simulink model "Agent_ZP_Mananger"  (R2018a)
settings: Solver=FixedStepAuto  StartTime=0.0  StopTime=Inf  FixedStep=0.0000001  RelTol=1e-3
(part 1 of 2)
settings Model: Creator=lenovo  LastModifiedBy=lenovo

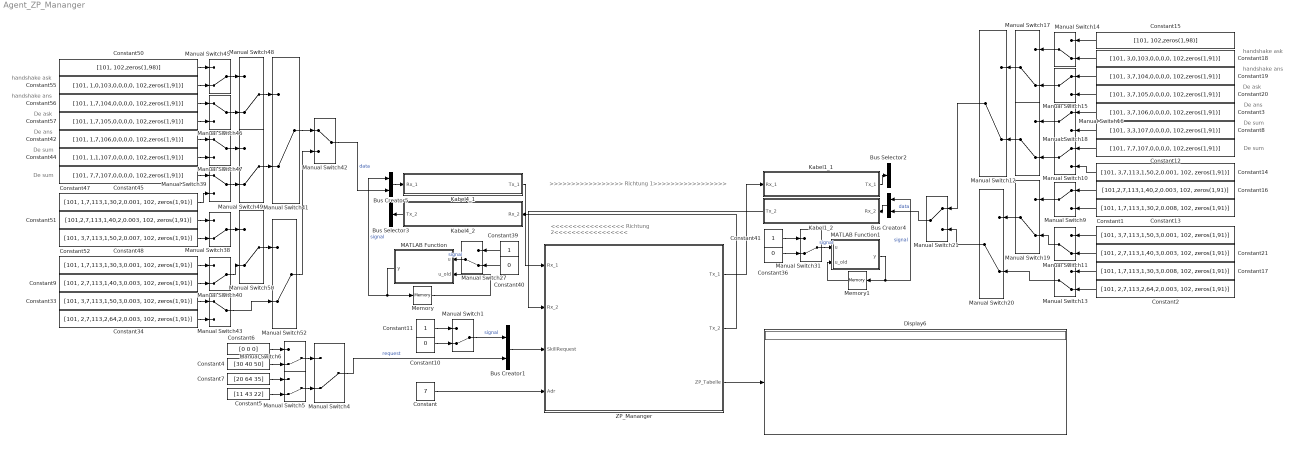
== system Agent_ZP_Mananger ==
  note: >>>>>>>>>>>>>>>>> Richtung 1>>>>>>>>>>>>>>>>>
  note: handshake ask
  note: De sum
  note: handshake ans
  note: De ask
  note: De ans
  note: De sum
  note: De ask
  note: De sum
  note: De ans
  note: handshake ans
  note: De sum
  note: handshake ask
  note: <<<<<<<<<<<<<<<<< Richtung 2<<<<<<<<<<<<<<<<<
  Bus Creator1 : BusCreator  Inputs=2
  Bus Creator4 : BusCreator  Inputs=2
  Bus Creator5 : BusCreator  Inputs=2
  Bus Selector2 : BusSelector  OutputSignals=signal,data
  Bus Selector3 : BusSelector  OutputSignals=signal,data
  Constant : Constant  Value=7  OutDataTypeStr=double
  Constant1 : Constant  Value=[101, 3,7,113,1,50,3,0.001, 102, zeros(1,91)]  OutDataTypeStr=double
  Constant10 : Constant  Value=0  OutDataTypeStr=boolean
  Constant11 : Constant  OutDataTypeStr=boolean
  Constant12 : Constant  Value=[101, 7,7,107,0,0,0,0, 102,zeros(1,91)]  OutDataTypeStr=double
  Constant13 : Constant  Value=[101, 1,7,113,1,30,2,0.008, 102, zeros(1,91)]  OutDataTypeStr=double
  Constant14 : Constant  Value=[101, 3,7,113,1,50,2,0.001, 102, zeros(1,91)]  OutDataTypeStr=double
  Constant15 : Constant  Value=[101, 102,zeros(1,98)]  OutDataTypeStr=double
  Constant16 : Constant  Value=[101,2,7,113,1,40,2,0.003, 102, zeros(1,91)]  OutDataTypeStr=double
  Constant17 : Constant  Value=[101, 1,7,113,1,30,3,0.008, 102, zeros(1,91)]  OutDataTypeStr=double
  Constant18 : Constant  Value=[101, 3,0,103,0,0,0,0, 102,zeros(1,91)]  OutDataTypeStr=double
  Constant19 : Constant  Value=[101, 3,7,104,0,0,0,0, 102,zeros(1,91)]  OutDataTypeStr=double
  Constant2 : Constant  Value=[101, 2,7,113,2,64,2,0.003, 102, zeros(1,91)]  OutDataTypeStr=double
  Constant20 : Constant  Value=[101, 3,7,105,0,0,0,0, 102,zeros(1,91)]  OutDataTypeStr=double
  Constant21 : Constant  Value=[101, 2,7,113,1,40,3,0.003, 102, zeros(1,91)]  OutDataTypeStr=double
  Constant3 : Constant  Value=[101, 3,7,106,0,0,0,0, 102,zeros(1,91)]  OutDataTypeStr=double
  Constant33 : Constant  Value=[101, 3,7,113,1,50,3,0.003, 102, zeros(1,91)]  OutDataTypeStr=double
  Constant34 : Constant  Value=[101, 2,7,113,2,64,2,0.003, 102, zeros(1,91)]  OutDataTypeStr=double
  Constant36 : Constant  Value=0  OutDataTypeStr=boolean
  Constant39 : Constant  OutDataTypeStr=boolean
  Constant4 : Constant  Value=[30 40 50]
  Constant40 : Constant  Value=0  OutDataTypeStr=boolean
  Constant41 : Constant  OutDataTypeStr=boolean
  Constant42 : Constant  Value=[101, 1,7,106,0,0,0,0, 102,zeros(1,91)]  OutDataTypeStr=double
  Constant44 : Constant  Value=[101, 1,1,107,0,0,0,0, 102,zeros(1,91)]  OutDataTypeStr=double
  Constant45 : Constant  Value=[101, 7,7,107,0,0,0,0, 102,zeros(1,91)]  OutDataTypeStr=double
  Constant47 : Constant  Value=[101, 1,7,113,1,30,2,0.001, 102, zeros(1,91)]  OutDataTypeStr=double
  Constant48 : Constant  Value=[101, 3,7,113,1,50,2,0.007, 102, zeros(1,91)]  OutDataTypeStr=double
  Constant5 : Constant  Value=[11 43 22]
  Constant50 : Constant  Value=[101, 102,zeros(1,98)]  OutDataTypeStr=double
  Constant51 : Constant  Value=[101,2,7,113,1,40,2,0.003, 102, zeros(1,91)]  OutDataTypeStr=double
  Constant52 : Constant  Value=[101, 1,7,113,1,30,3,0.001, 102, zeros(1,91)]  OutDataTypeStr=double
  Constant55 : Constant  Value=[101, 1,0,103,0,0,0,0, 102,zeros(1,91)]  OutDataTypeStr=double
  Constant56 : Constant  Value=[101, 1,7,104,0,0,0,0, 102,zeros(1,91)]  OutDataTypeStr=double
  Constant57 : Constant  Value=[101, 1,7,105,0,0,0,0, 102,zeros(1,91)]  OutDataTypeStr=double
  Constant6 : Constant  Value=[0 0 0]
  Constant7 : Constant  Value=[20 64 35]
  Constant8 : Constant  Value=[101, 3,3,107,0,0,0,0, 102,zeros(1,91)]  OutDataTypeStr=double
  Constant9 : Constant  Value=[101, 2,7,113,1,40,3,0.003, 102, zeros(1,91)]  OutDataTypeStr=double
  Display6 : Display
  Kabel1_1 : Subsystem  TreatAsAtomicUnit=on
  Kabel1_2 : Subsystem  TreatAsAtomicUnit=on
  Kabel4_1 : Subsystem  TreatAsAtomicUnit=on
  Kabel4_2 : Subsystem  TreatAsAtomicUnit=on
  MATLAB Function : MATLAB Function  TreatAsAtomicUnit=on  SystemSampleTime=0.00001
  MATLAB Function1 : MATLAB Function  TreatAsAtomicUnit=on  SystemSampleTime=0.00001
  Manual Switch{1,4..6,11..14,17..20,27,31,38,40..41,45,48..50,52} (22 alike) : ManualSwitch  CurrentSetting=0
  Manual Switch{9..10,15..16,21,39,42..43,46..47} (10 alike) : ManualSwitch
  Memory : Memory  InitialCondition=false
  Memory1 : Memory  InitialCondition=false
  ZP_Mananger : Subsystem
  wires:
  Constant4/1 -> Manual Switch6/2
  Constant7/1 -> Manual Switch5/1
  Constant6/1 -> Manual Switch6/1
  Constant5/1 -> Manual Switch5/2
  Manual Switch5/1 -> Manual Switch4/2
  Manual Switch6/1 -> Manual Switch4/1
  Constant40/1 -> Manual Switch27/2
  Kabel1_1/1(Tx_1) -> Bus Selector2/1
  MATLAB Function/1(y) -> Memory/1, Bus Creator5/1  "signal"
  Bus Creator5/1 -> Kabel4_1/1(Rx_1)
  Bus Creator4/1 -> Kabel1_2/1(Rx_2)
  Constant36/1 -> Manual Switch31/2
  Constant41/1 -> Manual Switch31/1
  Memory1/1 -> MATLAB Function1/2(u_old)
  Manual Switch31/1 -> MATLAB Function1/1(u)  "signal"
  Memory/1 -> MATLAB Function/2(u_old)
  Manual Switch27/1 -> MATLAB Function/1(u)  "signal"
  MATLAB Function1/1(y) -> Bus Creator4/1, Memory1/1  "signal"
  Constant39/1 -> Manual Switch27/1
  Kabel4_2/1(Tx_2) -> Bus Selector3/1
  Constant44/1 -> Manual Switch47/2
  Constant57/1 -> Manual Switch46/2
  Constant56/1 -> Manual Switch46/1
  Constant55/1 -> Manual Switch45/2
  Constant50/1 -> Manual Switch45/1
  Manual Switch52/1 -> Manual Switch42/2
  Manual Switch50/1 -> Manual Switch52/1
  Manual Switch47/1 -> Manual Switch49/1
  Manual Switch38/1 -> Manual Switch50/1
  Manual Switch43/1 -> Manual Switch52/2
  Manual Switch48/1 -> Manual Switch41/1
  Constant42/1 -> Manual Switch47/1
  Manual Switch39/1 -> Manual Switch49/2
  Manual Switch46/1 -> Manual Switch48/2
  Manual Switch49/1 -> Manual Switch41/2
  Manual Switch45/1 -> Manual Switch48/1
  Manual Switch41/1 -> Manual Switch42/1
  Constant45/1 -> Manual Switch39/1
  Manual Switch40/1 -> Manual Switch50/2
  Manual Switch42/1 -> Bus Creator5/2  "data"
  Manual Switch21/1 -> Bus Creator4/2  "data"
  Constant47/1 -> Manual Switch39/2
  Constant51/1 -> Manual Switch38/1
  Constant48/1 -> Manual Switch38/2
  Constant52/1 -> Manual Switch40/1
  Constant9/1 -> Manual Switch40/2
  Constant33/1 -> Manual Switch43/1
  Constant34/1 -> Manual Switch43/2
  Constant20/1 -> Manual Switch15/2
  Manual Switch10/1 -> Manual Switch18/2
  Constant3/1 -> Manual Switch16/1
  Constant1/1 -> Manual Switch11/1
  Manual Switch17/1 -> Manual Switch12/1
  Manual Switch16/1 -> Manual Switch18/1
  Manual Switch19/1 -> Manual Switch20/1
  Constant15/1 -> Manual Switch14/1
  Constant18/1 -> Manual Switch14/2
  Manual Switch15/1 -> Manual Switch17/2
  Manual Switch18/1 -> Manual Switch12/2
  Manual Switch14/1 -> Manual Switch17/1
  Manual Switch11/1 -> Manual Switch19/2
  Constant8/1 -> Manual Switch16/2
  Constant12/1 -> Manual Switch10/1
  Constant21/1 -> Manual Switch11/2
  Manual Switch9/1 -> Manual Switch19/1
  Constant2/1 -> Manual Switch13/2
  Constant19/1 -> Manual Switch15/1
  Manual Switch13/1 -> Manual Switch20/2
  Constant16/1 -> Manual Switch9/1
  Manual Switch12/1 -> Manual Switch21/1
  Manual Switch20/1 -> Manual Switch21/2
  Constant13/1 -> Manual Switch9/2
  Constant14/1 -> Manual Switch10/2
  Constant17/1 -> Manual Switch13/1
  Kabel4_1/1(Tx_1) -> ZP_Mananger/1(Rx_1)
  Kabel1_2/1(Tx_2) -> ZP_Mananger/2(Rx_2)
  Constant/1 -> ZP_Mananger/4(Adr)
  ZP_Mananger/1(Tx_1) -> Kabel1_1/1(Rx_1)
  ZP_Mananger/2(Tx_2) -> Kabel4_2/1(Rx_2)
  Manual Switch1/1 -> Bus Creator1/1  "signal"
  Manual Switch4/1 -> Bus Creator1/2  "request"
  Bus Creator1/1 -> ZP_Mananger/3(SkillRequest)
  Constant10/1 -> Manual Switch1/2
  Constant11/1 -> Manual Switch1/1
  ZP_Mananger/3(ZP_Tabelle) -> Display6/1

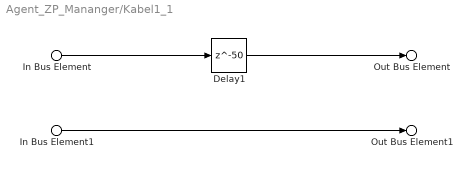
== system Agent_ZP_Mananger/Kabel1_1 ==
  In Bus Element : Inport  PortName=Rx_1  Element=signal
  In Bus Element1 : Inport  PortName=Rx_1  Element=data
  Delay1 : Delay  DelayLength=50
  Out Bus Element : Outport  PortName=Tx_1  Element=signal
  Out Bus Element1 : Outport  PortName=Tx_1  Element=data
  wires:
  In Bus Element/1 -> Delay1/1
  Delay1/1 -> Out Bus Element/1
  In Bus Element1/1 -> Out Bus Element1/1

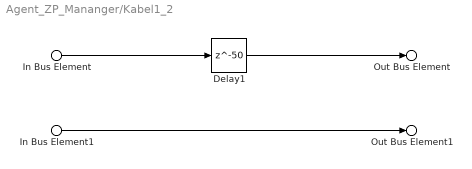
== system Agent_ZP_Mananger/Kabel1_2 ==
  In Bus Element : Inport  PortName=Rx_2  Element=signal
  In Bus Element1 : Inport  PortName=Rx_2  Element=data
  Delay1 : Delay  DelayLength=50
  Out Bus Element : Outport  PortName=Tx_2  Element=signal
  Out Bus Element1 : Outport  PortName=Tx_2  Element=data
  wires:
  In Bus Element/1 -> Delay1/1
  Delay1/1 -> Out Bus Element/1
  In Bus Element1/1 -> Out Bus Element1/1

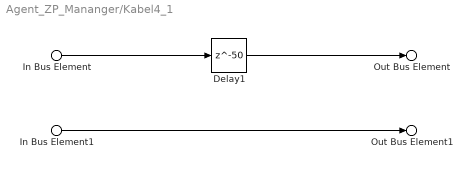
== system Agent_ZP_Mananger/Kabel4_1 ==
  In Bus Element : Inport  PortName=Rx_1  Element=signal
  In Bus Element1 : Inport  PortName=Rx_1  Element=data
  Delay1 : Delay  DelayLength=50
  Out Bus Element : Outport  PortName=Tx_1  Element=signal
  Out Bus Element1 : Outport  PortName=Tx_1  Element=data
  wires:
  In Bus Element/1 -> Delay1/1
  Delay1/1 -> Out Bus Element/1
  In Bus Element1/1 -> Out Bus Element1/1

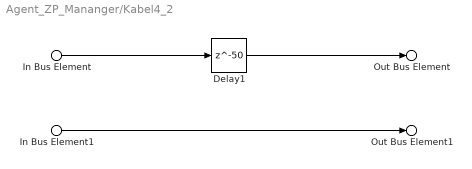
== system Agent_ZP_Mananger/Kabel4_2 ==
  In Bus Element : Inport  PortName=Rx_2  Element=signal
  In Bus Element1 : Inport  PortName=Rx_2  Element=data
  Delay1 : Delay  DelayLength=50
  Out Bus Element : Outport  PortName=Tx_2  Element=signal
  Out Bus Element1 : Outport  PortName=Tx_2  Element=data
  wires:
  In Bus Element/1 -> Delay1/1
  Delay1/1 -> Out Bus Element/1
  In Bus Element1/1 -> Out Bus Element1/1

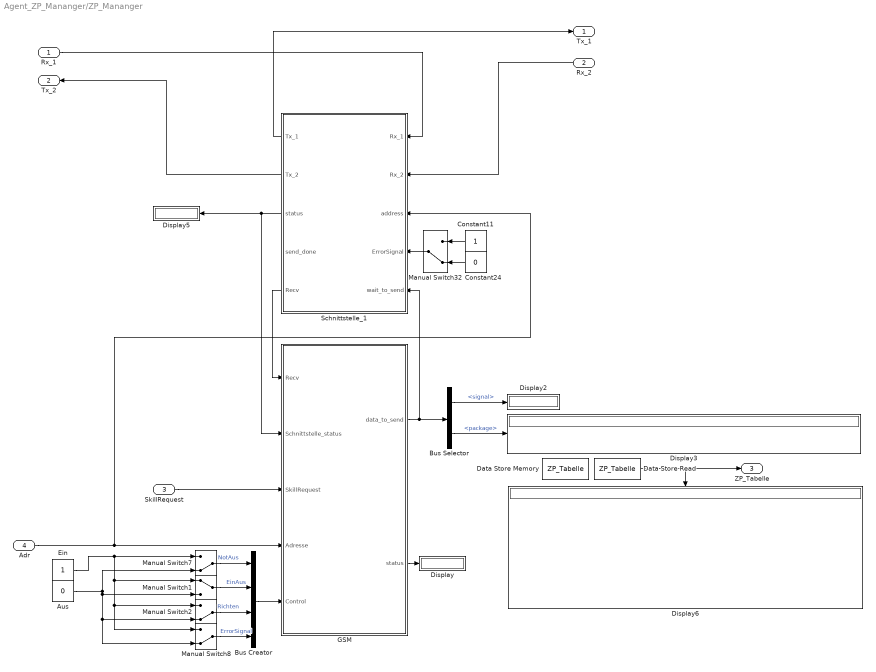
== system Agent_ZP_Mananger/ZP_Mananger ==
  Rx_1 : Inport
  Rx_2 : Inport  Port=2
  SkillRequest : Inport  Port=3
  Adr : Inport  Port=4
  Aus : Constant  Value=0  OutDataTypeStr=boolean
  Bus Creator : BusCreator  Inputs=4
  Bus Selector : BusSelector  OutputSignals=signal,package
  Constant11 : Constant  OutDataTypeStr=boolean
  Constant24 : Constant  Value=0  OutDataTypeStr=boolean
  Data Store Memory : DataStoreMemory  DataStoreName=ZP_Tabelle  ReadBeforeWriteMsg=warning  WriteAfterWriteMsg=warning  WriteAfterReadMsg=warning  InitialValue=zeros(10,7)  ShowAdditionalParam=off  OutDataTypeStr=double  Dimensions=[10 7]
  Data Store Read : DataStoreRead  DataStoreName=ZP_Tabelle
  Display{,2..3,5..6} (5 alike) : Display
  Ein : Constant  OutDataTypeStr=boolean
  "GSM " : Subsystem
  Manual Switch1 : ManualSwitch
  Manual Switch{2,7..8,32} (4 alike) : ManualSwitch  CurrentSetting=0
  Schnittstelle_1 : Subsystem
  Tx_1 : Outport
  Tx_2 : Outport  Port=2
  ZP_Tabelle : Outport  Port=3
  wires:
  Bus Selector/1 -> Display2/1  "<signal>"
  Ein/1 -> Manual Switch7/1, Manual Switch1/1, Manual Switch2/1, Manual Switch8/1
  Data Store Read/1 -> ZP_Tabelle/1, Display6/1
  Schnittstelle_1/5(Recv) -> "GSM "/1(Recv)
  Aus/1 -> Manual Switch7/2, Manual Switch1/2, Manual Switch2/2, Manual Switch8/2
  Manual Switch32/1 -> Schnittstelle_1/4(ErrorSignal)
  Manual Switch1/1 -> Bus Creator/2  "EinAus"
  Manual Switch8/1 -> Bus Creator/4  "ErrorSignal"
  Bus Selector/2 -> Display3/1  "<package>"
  "GSM "/2(status) -> Display/1
  Schnittstelle_1/3(status) -> "GSM "/2(Schnittstelle_status), Display5/1
  Manual Switch2/1 -> Bus Creator/3  "Richten"
  "GSM "/1(data_to_send) -> Bus Selector/1, Schnittstelle_1/5(wait_to_send)
  Bus Creator/1 -> "GSM "/5(Control)
  Constant24/1 -> Manual Switch32/2
  Constant11/1 -> Manual Switch32/1
  Manual Switch7/1 -> Bus Creator/1  "NotAus"
  Schnittstelle_1/1(Tx_1) -> Tx_1/1
  Rx_1/1 -> Schnittstelle_1/1(Rx_1)
  Rx_2/1 -> Schnittstelle_1/2(Rx_2)
  Schnittstelle_1/2(Tx_2) -> Tx_2/1
  Adr/1 -> Schnittstelle_1/3(address), "GSM "/4(Adresse)
  SkillRequest/1 -> "GSM "/3(SkillRequest)

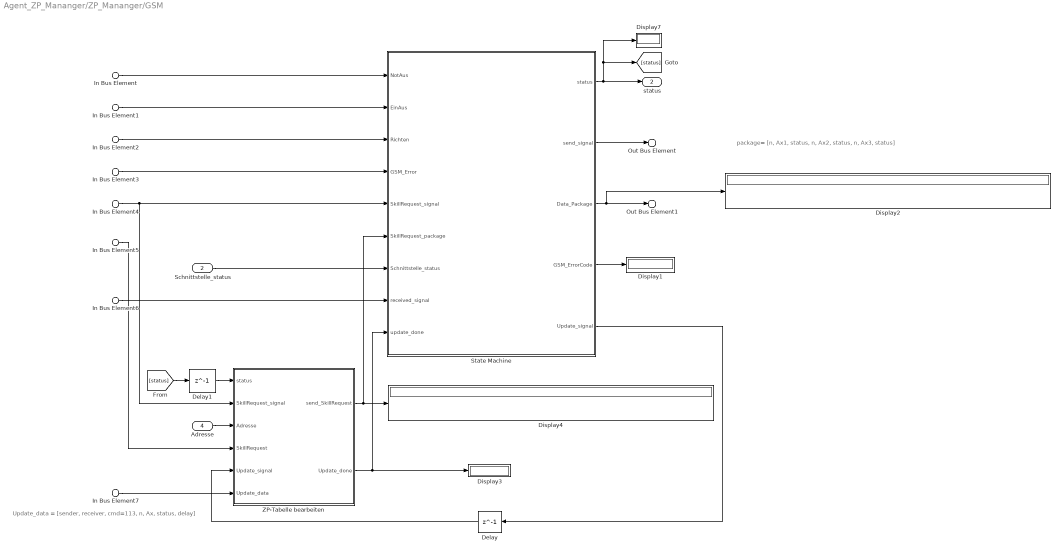
== system Agent_ZP_Mananger/ZP_Mananger/GSM  ==
  note: package= [n, Ax1, status, n, Ax2, status, n, Ax3, status]
  note: Update_data = [sender, receiver, cmd=113, n, Ax, status, delay]
  In Bus Element6 : Inport  PortName=Recv  Element=signal
  In Bus Element7 : Inport  PortName=Recv  Element=package
  Schnittstelle_status : Inport  Port=2  OutDataTypeStr=double
  In Bus Element4 : Inport  Port=3  PortName=SkillRequest  Element=signal
  In Bus Element5 : Inport  Port=3  PortName=SkillRequest  Element=request
  Adresse : Inport  Port=4
  In Bus Element : Inport  Port=5  PortName=Control  Element=NotAus
  In Bus Element1 : Inport  Port=5  PortName=Control  Element=EinAus
  In Bus Element2 : Inport  Port=5  PortName=Control  Element=Richten
  In Bus Element3 : Inport  Port=5  PortName=Control  Element=ErrorSignal
  Delay : Delay  DelayLength=1
  Delay1 : Delay  DelayLength=1
  Display{1..4,7} (5 alike) : Display
  State Machine : Stateflow chart  TreatAsAtomicUnit=on
  ZP-Tabelle bearbeiten : Subsystem
  Out Bus Element : Outport  PortName=data_to_send  Element=signal
  Out Bus Element1 : Outport  PortName=data_to_send  Element=package
  status : Outport  Port=2
  wires:
  In Bus Element6/1 -> State Machine/8(received_signal)
  In Bus Element2/1 -> State Machine/3(Richten)
  State Machine/1(status) -> Display7/1, [status], status/1
  In Bus Element/1 -> State Machine/1(NotAus)
  In Bus Element1/1 -> State Machine/2(EinAus)
  Schnittstelle_status/1 -> State Machine/7(Schnittstelle_status)
  State Machine/4(GSM_ErrorCode) -> Display1/1
  In Bus Element4/1 -> State Machine/5(SkillRequest_signal), ZP-Tabelle bearbeiten/2(SkillRequest_signal)
  In Bus Element5/1 -> ZP-Tabelle bearbeiten/4(SkillRequest)
  In Bus Element3/1 -> State Machine/4(GSM_Error)
  State Machine/2(send_signal) -> Out Bus Element/1
  State Machine/3(Data_Package) -> Out Bus Element1/1, Display2/1
  In Bus Element7/1 -> ZP-Tabelle bearbeiten/6(Update_data)
  ZP-Tabelle bearbeiten/1(send_SkillRequest) -> State Machine/6(SkillRequest_package), Display4/1
  ZP-Tabelle bearbeiten/2(Update_done) -> Display3/1, State Machine/9(update_done)
  State Machine/5(Update_signal) -> Delay/1
  Delay/1 -> ZP-Tabelle bearbeiten/5(Update_signal)
  Adresse/1 -> ZP-Tabelle bearbeiten/3(Adresse)
  [status] -> Delay1/1
  Delay1/1 -> ZP-Tabelle bearbeiten/1(status)

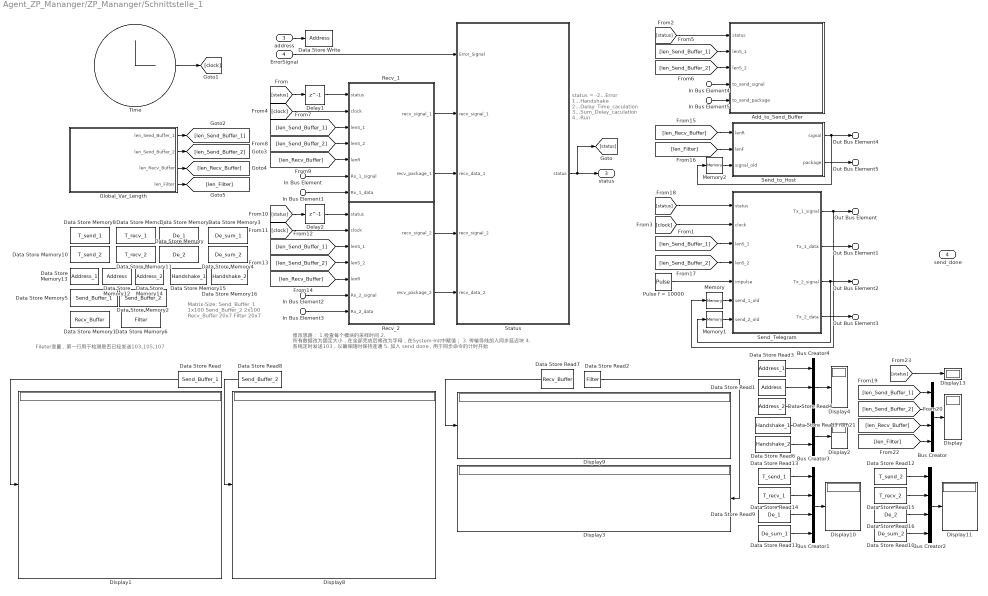
== system Agent_ZP_Mananger/ZP_Mananger/Schnittstelle_1 ==
  note: Fileter变量，第一行用于检测是否已经发送103,105,107
  note: 修改思路：
      | 1.检查每个模块的采样时间
      | 2. 所有数据改为固定大小，在全部完成后修改为字母，在System-Init中赋值；
      | 3. 传输导线加入同步延迟块
      | 4. 系统定时发送103，以确保随时保持连通
      | 5. 加入 send done，用于同步命令的计时开始
  note: status =
      | -2...Error
      |  1...Handshake
      |  2...Delay_Time_caculation
      |  3...Sum_Delay_caculation
      |  4...Run
  note: Matrix-Size:
      | Send_Buffer_1	1x100
      | Send_Buffer_2	2x100
      | Recv_Buffer		20x7
      | Filter			20x7
  In Bus Element : Inport  PortName=Rx_1  Element=signal
  In Bus Element1 : Inport  PortName=Rx_1  Element=data
  In Bus Element2 : Inport  Port=2  PortName=Rx_2  Element=signal
  In Bus Element3 : Inport  Port=2  PortName=Rx_2  Element=data
  address : Inport  Port=3
  ErrorSignal : Inport  Port=4
  In Bus Element4 : Inport  Port=5  PortName=wait_to_send  Element=signal
  In Bus Element5 : Inport  Port=5  PortName=wait_to_send  Element=package
  Add_to_Send_Buffer : MATLAB Function  TreatAsAtomicUnit=on  SystemSampleTime=0.00001
  Bus Creator : BusCreator  Inputs=4
  Bus Creator1 : BusCreator  Inputs=4
  Bus Creator2 : BusCreator  Inputs=4
  Bus Creator3 : BusCreator  Inputs=2
  Bus Creator4 : BusCreator  Inputs=3
  Data Store Memory : DataStoreMemory  DataStoreName=De_2  ReadBeforeWriteMsg=warning  WriteAfterWriteMsg=warning  WriteAfterReadMsg=warning  ShowAdditionalParam=off  OutDataTypeStr=double  Dimensions=1
  Data Store Memory1 : DataStoreMemory  DataStoreName=Recv_Buffer  ReadBeforeWriteMsg=warning  WriteAfterWriteMsg=warning  WriteAfterReadMsg=warning  InitialValue=zeros(20,7)  VectorParams1D=off  ShowAdditionalParam=off  OutDataTypeStr=double  Dimensions=[20,7]
  Data Store Memory10 : DataStoreMemory  DataStoreName=T_send_2  ReadBeforeWriteMsg=warning  WriteAfterWriteMsg=warning  WriteAfterReadMsg=warning  ShowAdditionalParam=off  OutDataTypeStr=double  Dimensions=1
  Data Store Memory11 : DataStoreMemory  DataStoreName=T_recv_2  ReadBeforeWriteMsg=warning  WriteAfterWriteMsg=warning  WriteAfterReadMsg=warning  ShowAdditionalParam=off  OutDataTypeStr=double  Dimensions=1
  Data Store Memory12 : DataStoreMemory  DataStoreName=Address  ReadBeforeWriteMsg=warning  WriteAfterWriteMsg=warning  WriteAfterReadMsg=warning  ShowAdditionalParam=off  OutDataTypeStr=double  Dimensions=1
  Data Store Memory13 : DataStoreMemory  DataStoreName=Address_1  ReadBeforeWriteMsg=warning  WriteAfterWriteMsg=warning  WriteAfterReadMsg=warning  ShowAdditionalParam=off  OutDataTypeStr=double  Dimensions=1
  Data Store Memory14 : DataStoreMemory  DataStoreName=Address_2  ReadBeforeWriteMsg=warning  WriteAfterWriteMsg=warning  WriteAfterReadMsg=warning  ShowAdditionalParam=off  OutDataTypeStr=double  Dimensions=1
  Data Store Memory15 : DataStoreMemory  DataStoreName=Handshake_1  ReadBeforeWriteMsg=warning  WriteAfterWriteMsg=warning  WriteAfterReadMsg=warning  InitialValue=false  ShowAdditionalParam=off  OutDataTypeStr=boolean
  Data Store Memory16 : DataStoreMemory  DataStoreName=Handshake_2  ReadBeforeWriteMsg=warning  WriteAfterWriteMsg=warning  WriteAfterReadMsg=warning  InitialValue=false  ShowAdditionalParam=off  OutDataTypeStr=boolean
  Data Store Memory2 : DataStoreMemory  DataStoreName=Send_Buffer_2  ReadBeforeWriteMsg=warning  WriteAfterWriteMsg=warning  WriteAfterReadMsg=warning  InitialValue=[101, 102, zeros(1,98)]  VectorParams1D=off  ShowAdditionalParam=off  OutDataTypeStr=double  Dimensions=[1,100]
  Data Store Memory3 : DataStoreMemory  DataStoreName=De_sum_1  ReadBeforeWriteMsg=warning  WriteAfterWriteMsg=warning  WriteAfterReadMsg=warning  ShowAdditionalParam=off  OutDataTypeStr=double  Dimensions=1
  Data Store Memory4 : DataStoreMemory  DataStoreName=De_sum_2  ReadBeforeWriteMsg=warning  WriteAfterWriteMsg=warning  WriteAfterReadMsg=warning  ShowAdditionalParam=off  OutDataTypeStr=double  Dimensions=1
  Data Store Memory5 : DataStoreMemory  DataStoreName=Send_Buffer_1  ReadBeforeWriteMsg=warning  WriteAfterWriteMsg=warning  WriteAfterReadMsg=warning  InitialValue=[101, 102, zeros(1,98)]  VectorParams1D=off  ShowAdditionalParam=off  OutDataTypeStr=double  Dimensions=[1,100]
  Data Store Memory6 : DataStoreMemory  DataStoreName=Filter  ReadBeforeWriteMsg=warning  WriteAfterWriteMsg=warning  WriteAfterReadMsg=warning  InitialValue=zeros(20,7)  VectorParams1D=off  ShowAdditionalParam=off  OutDataTypeStr=double  Dimensions=[20,7]
  Data Store Memory7 : DataStoreMemory  DataStoreName=De_1  ReadBeforeWriteMsg=warning  WriteAfterWriteMsg=warning  WriteAfterReadMsg=warning  ShowAdditionalParam=off  OutDataTypeStr=double  Dimensions=1
  Data Store Memory8 : DataStoreMemory  DataStoreName=T_send_1  ReadBeforeWriteMsg=warning  WriteAfterWriteMsg=warning  WriteAfterReadMsg=warning  ShowAdditionalParam=off  OutDataTypeStr=double  Dimensions=1
  Data Store Memory9 : DataStoreMemory  DataStoreName=T_recv_1  ReadBeforeWriteMsg=warning  WriteAfterWriteMsg=warning  WriteAfterReadMsg=warning  ShowAdditionalParam=off  OutDataTypeStr=double  Dimensions=1
  Data Store Read : DataStoreRead  DataStoreName=Send_Buffer_1
  Data Store Read1 : DataStoreRead  DataStoreName=Address
  Data Store Read10 : DataStoreRead  DataStoreName=De_sum_2
  Data Store Read11 : DataStoreRead  DataStoreName=De_sum_1
  Data Store Read12 : DataStoreRead  DataStoreName=T_send_2
  Data Store Read13 : DataStoreRead  DataStoreName=T_send_1
  Data Store Read14 : DataStoreRead  DataStoreName=T_recv_1
  Data Store Read15 : DataStoreRead  DataStoreName=T_recv_2
  Data Store Read16 : DataStoreRead  DataStoreName=De_2
  Data Store Read2 : DataStoreRead  DataStoreName=Filter
  Data Store Read3 : DataStoreRead  DataStoreName=Address_1
  Data Store Read4 : DataStoreRead  DataStoreName=Address_2
  Data Store Read5 : DataStoreRead  DataStoreName=Handshake_1
  Data Store Read6 : DataStoreRead  DataStoreName=Handshake_2
  Data Store Read7 : DataStoreRead  DataStoreName=Recv_Buffer
  Data Store Read8 : DataStoreRead  DataStoreName=Send_Buffer_2
  Data Store Read9 : DataStoreRead  DataStoreName=De_1
  Data Store Write : DataStoreWrite  DataStoreName=Address
  Delay1 : Delay  DelayLength=1
  Delay2 : Delay  DelayLength=1
  Display{,1..4,8..11,13} (10 alike) : Display
  Global_Var_Length : MATLAB Function  TreatAsAtomicUnit=on
  Memory : Memory  InitialCondition=false
  Memory1 : Memory  InitialCondition=false
  Memory2 : Memory  InitialCondition=false
  Pulse f = 10000 : DiscretePulseGenerator  PulseType=Time based  Amplitude=true  Period=1/1000  PulseWidth=30
  Recv_1 : MATLAB Function  TreatAsAtomicUnit=on  SystemSampleTime=0.00001
  Recv_2 : MATLAB Function  TreatAsAtomicUnit=on  SystemSampleTime=0.00001
  Send_Telegram : MATLAB Function  TreatAsAtomicUnit=on  SystemSampleTime=0.00001
  Send_to_Host : MATLAB Function  TreatAsAtomicUnit=on  SystemSampleTime=0.00001
  Status : Stateflow chart  TreatAsAtomicUnit=on  SystemSampleTime=0.0000001
  Time : Clock
  Out Bus Element : Outport  PortName=Tx_1  Element=signal
  Out Bus Element1 : Outport  PortName=Tx_1  Element=data
  Out Bus Element2 : Outport  Port=2  PortName=Tx_2  Element=signal
  Out Bus Element3 : Outport  Port=2  PortName=Tx_2  Element=data
  status : Outport  Port=3
  send_done : Outport  Port=4
  Out Bus Element4 : Outport  Port=5  PortName=Recv  Element=signal
  Out Bus Element5 : Outport  Port=5  PortName=Recv  Element=package
  wires:
  ErrorSignal/1 -> Status/1(Error_Signal)
  Status/1(status) -> [status], status/1
  Pulse f = 10000/1 -> Send_Telegram/5(impulse)
  In Bus Element1/1 -> Recv_1/7(Rx_1_data)
  In Bus Element/1 -> Recv_1/6(Rx_1_signal)
  Send_Telegram/1(Tx_1_signal) -> Memory/1, Out Bus Element/1
  Send_Telegram/3(Tx_2_signal) -> Memory1/1, Out Bus Element2/1
  Memory1/1 -> Send_Telegram/7(send_2_old)
  Memory/1 -> Send_Telegram/6(send_1_old)
  [status] -> Delay1/1
  Time/1 -> [clock]
  [clock] -> Recv_1/2(clock)
  Send_to_Host/1(signal) -> Out Bus Element4/1, Memory2/1
  address/1 -> Data Store Write/1
  Global_Var_Length/1(len_Send_Buffer_1) -> [len_Send_Buffer_1]
  Global_Var_Length/2(len_Send_Buffer_2) -> [len_Send_Buffer_2]
  Global_Var_Length/3(len_Recv_Buffer) -> [len_Recv_Buffer]
  Global_Var_Length/4(len_Filter) -> [len_Filter]
  [len_Send_Buffer_1] -> Recv_1/3(lenS_1)
  [len_Send_Buffer_2] -> Recv_1/4(lenS_2)
  [len_Recv_Buffer] -> Recv_1/5(lenR)
  In Bus Element2/1 -> Recv_2/6(Rx_2_signal)
  In Bus Element3/1 -> Recv_2/7(Rx_2_data)
  [status] -> Delay2/1
  [len_Recv_Buffer] -> Recv_2/5(lenR)
  [len_Send_Buffer_1] -> Recv_2/3(lenS_1)
  [clock] -> Recv_2/2(clock)
  [len_Send_Buffer_2] -> Recv_2/4(lenS_2)
  Delay1/1 -> Recv_1/1(status)
  Delay2/1 -> Recv_2/1(status)
  Recv_1/1(recv_signal_1) -> Status/2(recv_signal_1)
  Recv_1/2(recv_package_1) -> Status/3(recv_data_1)
  Recv_2/1(recv_signal_2) -> Status/4(recv_signal_2)
  Recv_2/2(recv_package_2) -> Status/5(recv_data_2)
  [len_Recv_Buffer] -> Send_to_Host/1(lenR)
  [len_Filter] -> Send_to_Host/2(lenF)
  Send_Telegram/4(Tx_2_data) -> Out Bus Element3/1
  [len_Send_Buffer_1] -> Send_Telegram/3(lenS_1)
  [len_Send_Buffer_2] -> Send_Telegram/4(lenS_2)
  [clock] -> Send_Telegram/2(clock)
  [status] -> Send_Telegram/1(status)
  Send_Telegram/2(Tx_1_data) -> Out Bus Element1/1
  [len_Send_Buffer_1] -> Add_to_Send_Buffer/2(lenS_1)
  [len_Send_Buffer_2] -> Add_to_Send_Buffer/3(lenS_2)
  In Bus Element4/1 -> Add_to_Send_Buffer/4(to_send_signal)
  In Bus Element5/1 -> Add_to_Send_Buffer/5(to_send_package)
  [status] -> Add_to_Send_Buffer/1(status)
  Memory2/1 -> Send_to_Host/3(signal_old)
  Bus Creator/1 -> Display/1
  [len_Send_Buffer_1] -> Bus Creator/1
  [len_Send_Buffer_2] -> Bus Creator/2
  [len_Recv_Buffer] -> Bus Creator/3
  [len_Filter] -> Bus Creator/4
  Data Store Read/1 -> Display1/1
  Data Store Read2/1 -> Display3/1
  Data Store Read8/1 -> Display8/1
  Data Store Read7/1 -> Display9/1
  Data Store Read13/1 -> Bus Creator1/1
  Data Store Read14/1 -> Bus Creator1/2
  Data Store Read11/1 -> Bus Creator1/4
  Data Store Read9/1 -> Bus Creator1/3
  Bus Creator1/1 -> Display10/1
  Data Store Read12/1 -> Bus Creator2/1
  Data Store Read15/1 -> Bus Creator2/2
  Bus Creator2/1 -> Display11/1
  Data Store Read16/1 -> Bus Creator2/3
  Data Store Read10/1 -> Bus Creator2/4
  [status] -> Display13/1
  Send_to_Host/2(package) -> Out Bus Element5/1
  Data Store Read5/1 -> Bus Creator3/1
  Data Store Read6/1 -> Bus Creator3/2
  Data Store Read4/1 -> Bus Creator4/3
  Data Store Read1/1 -> Bus Creator4/2
  Data Store Read3/1 -> Bus Creator4/1
  Bus Creator3/1 -> Display2/1
  Bus Creator4/1 -> Display4/1

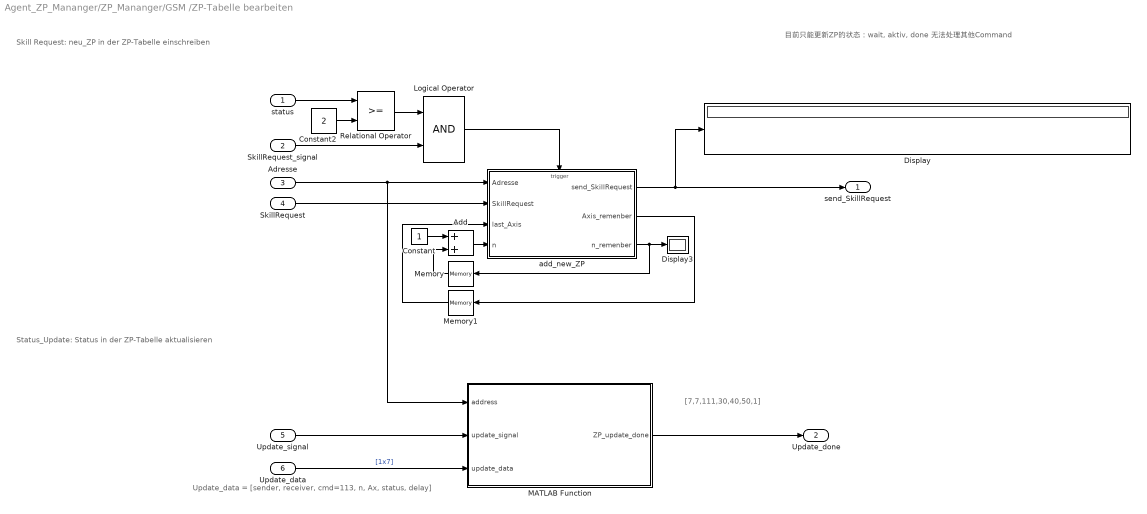
== system Agent_ZP_Mananger/ZP_Mananger/GSM /ZP-Tabelle bearbeiten ==
  note: Update_data = [sender, receiver, cmd=113, n, Ax, status, delay]
  note: Skill Request: neu_ZP in der ZP-Tabelle einschreiben
  note: Status_Update: Status in der ZP-Tabelle aktualisieren
  note: 目前只能更新ZP的状态：wait, aktiv, done
      | 无法处理其他Command
  note: [7,7,111,30,40,50,1]
  status : Inport
  SkillRequest_signal : Inport  Port=2  OutDataTypeStr=boolean
  Adresse : Inport  Port=3
  SkillRequest : Inport  Port=4  OutDataTypeStr=double
  Update_signal : Inport  Port=5  OutDataTypeStr=boolean
  Update_data : Inport  Port=6  OutDataTypeStr=double
  Add : Sum
  Constant : Constant
  Constant2 : Constant  Value=2  OutDataTypeStr=double
  Display : Display
  Display3 : Display
  Logical Operator : Logic  AllPortsSameDT=off  OutDataTypeStr=boolean
  MATLAB Function : MATLAB Function  TreatAsAtomicUnit=on
  Memory : Memory
  Memory1 : Memory  InitialCondition=[0 0 0]
  Relational Operator : RelationalOperator  OutDataTypeStr=boolean  RndMeth=Simplest
  add_new_ZP : Subsystem
  send_SkillRequest : Outport
  Update_done : Outport  Port=2  OutDataTypeStr=boolean
  wires:
  Memory1/1 -> add_new_ZP/3(last_Axis)
  add_new_ZP/2(Axis_remenber) -> Memory1/1
  SkillRequest/1 -> add_new_ZP/2(SkillRequest)
  Update_signal/1 -> MATLAB Function/2(update_signal)
  Add/1 -> add_new_ZP/4(n)
  Update_data/1 -> MATLAB Function/3(update_data)  "[1x7]"
  MATLAB Function/1(ZP_update_done) -> Update_done/1
  Constant/1 -> Add/1
  SkillRequest_signal/1 -> Logical Operator/2
  Memory/1 -> Add/2
  add_new_ZP/3(n_remenber) -> Memory/1, Display3/1
  add_new_ZP/1(send_SkillRequest) -> Display/1, send_SkillRequest/1
  Relational Operator/1 -> Logical Operator/1
  Constant2/1 -> Relational Operator/2
  status/1 -> Relational Operator/1
  Logical Operator/1 -> add_new_ZP/Trigger
  Adresse/1 -> MATLAB Function/1(address), add_new_ZP/1(Adresse)

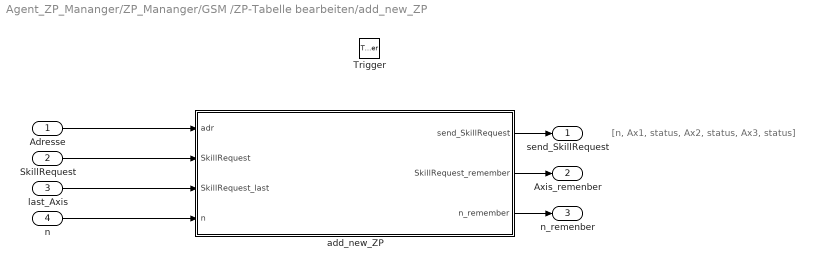
== system Agent_ZP_Mananger/ZP_Mananger/GSM /ZP-Tabelle bearbeiten/add_new_ZP ==
  note: [n, Ax1, status, Ax2, status, Ax3, status]
  Adresse : Inport
  SkillRequest : Inport  Port=2
  last_Axis : Inport  Port=3
  n : Inport  Port=4
  Trigger : TriggerPort  VariantControl=Variant  PortDimensions=1
  add_new_ZP : MATLAB Function  TreatAsAtomicUnit=on
  send_SkillRequest : Outport
  Axis_remenber : Outport  Port=2
  n_remenber : Outport  Port=3
  wires:
  n/1 -> add_new_ZP/4(n)
  SkillRequest/1 -> add_new_ZP/2(SkillRequest)
  add_new_ZP/1(send_SkillRequest) -> send_SkillRequest/1
  last_Axis/1 -> add_new_ZP/3(SkillRequest_last)
  add_new_ZP/3(n_remember) -> n_remenber/1
  add_new_ZP/2(SkillRequest_remember) -> Axis_remenber/1
  Adresse/1 -> add_new_ZP/1(adr)

== matlab function Agent_ZP_Mananger/ZP_Mananger/GSM /ZP-Tabelle bearbeiten/add_new_ZP/add_new_ZP ==
  data: adr input; SkillRequest input; SkillRequest_last input; n input; send_SkillRequest output double; SkillRequest_remember output; n_remember output; ZP_Tabelle data_store_memory
% neu SkillRequest in ZP-Tabelle eintragen
% Sendpackage erstellen

function [send_SkillRequest, SkillRequest_remember, n_remember] = add_new_ZP(adr, SkillRequest, SkillRequest_last, n)

global ZP_Tabelle

if ~isequal(SkillRequest,SkillRequest_last)   % same position filtern
    X = min(find(ZP_Tabelle(:,1)==0,1));      % find the first free line
    if ~isempty(X)
        ZP_Tabelle(X,:) = [n, SkillRequest(1), 1, SkillRequest(2), 1, SkillRequest(3), 1];  % add new ZP in the ZP-Tabelle
        send_SkillRequest = [adr,1,111,n,SkillRequest(1),1,0, adr,2,111,n,SkillRequest(2),1,0, adr,3,111,n,SkillRequest(3),1,0]; % create new ZP package
        n_remember = n;
    end
else
    send_SkillRequest = zeros(1,21);
    n_remember = n-1;
end

SkillRequest_remember = SkillRequest;
end

== stateflow chart Agent_ZP_Mananger/ZP_Mananger/GSM /State Machine ==
  settings: executeAtInitialization=1
  state Off
    entry: status = 0;
  state Error
    entry: status = -2;
  state Init
    entry: status = 1;
  state Run
    state Send_ZP
      entry:	status = 3;
      Data_Package = SkillRequest_package;
      send_signal = true;
    state Stand_By
      entry: status = 2;
    state ZP_Status_Update
      entry:	status = 4;
      Update_signal = received_signal;
    note: ZP_Status_Update = [address, command, n, Ax, status]
    note: received_package = [address, command, n, Ax, status]
    (default) -> Stand_By
    Stand_By -> Send_ZP [order 1] : [SkillRequest_signal]
    Send_ZP -> Stand_By : [~SkillRequest_signal]{send_signal=false;}
    ZP_Status_Update -> Stand_By : [update_done && ~received_signal]{Update_signal=false;}
    Stand_By -> ZP_Status_Update [order 2] : [received_signal && ~update_done]
  (default) -> Off
  Error -> Off [order 1] : [~EinAus]
  Off -> Error [order 2] : [EinAus && NotAus]
  Init -> Off [order 3] : [~EinAus]
  Off -> Init [order 1] : [EinAus && ~NotAus]
  Error -> Init [order 2] : [~GSM_Error && Richten] {GSM_ErrorCode=0;}
  Init -> Error [order 1] : [GSM_Error || NotAus]{GSM_ErrorCode=status}
  Run -> Init [order 2] : [Schnittstelle_status~=4 && ~GSM_Error]
  Init -> Run [order 2] : [Schnittstelle_status==4]
  Run -> Error [order 1] : [GSM_Error || NotAus]{GSM_ErrorCode=status}
  data: NotAus input boolean; EinAus input boolean; Richten input boolean; GSM_Error input boolean; SkillRequest_signal input boolean; SkillRequest_package input double; Schnittstelle_status input double; status output double; send_signal output boolean; received_signal input boolean; update_done input boolean; Data_Package output double; GSM_ErrorCode output double; Update_signal output boolean size=1

== matlab function Agent_ZP_Mananger/ZP_Mananger/GSM /ZP-Tabelle bearbeiten/MATLAB Function ==
  data: address input; update_signal input boolean; update_data input double size=7; ZP_update_done output boolean; ZP_Tabelle data_store_memory
%ZP_to_update = [address, command, n, Ax, status]

function ZP_update_done  = Status_Update(address, update_signal, update_data)

global ZP_Tabelle

if (update_signal && (update_data(2) == address))
    
    Y = 2 * update_data(1) + 1;             % Matrix-Index berechnen
    n = update_data(4);                     % ZP_n
    position = update_data(5);
    status = update_data(6);
    
    X = find(ZP_Tabelle(:,1)==n,1);	%ZP_N bestimmen
    if (~isempty(X) && isequal(ZP_Tabelle(X(1),Y-1),position))
        if ((status == -2) || ZP_Tabelle(X(1),Y) <= status)
            ZP_Tabelle(X(1),Y) = status;
        end
    end
    ZP_update_done = true;
    
else
    ZP_update_done = false;
    
end

end

== matlab function Agent_ZP_Mananger/MATLAB Function ==
  data: u input; y output; u_old input
function y  = fcn(u,u_old)

if u_old
    y = false;
else
    y = u;
end
end

== matlab function Agent_ZP_Mananger/MATLAB Function1 ==
  data: u input; y output; u_old input
function y  = fcn(u,u_old)

if u_old
    y = false;
else
    y = u;
end
end

== matlab function Agent_ZP_Mananger/ZP_Mananger/Schnittstelle_1/Add_to_Send_Buffer ==
  data: Send_Buffer_1 data_store_memory; Send_Buffer_2 data_store_memory; Address data_store_memory; status input; lenS_1 input; lenS_2 input; to_send_signal input; to_send_package input; Address_1 data_store_memory; Address_2 data_store_memory; Handshake_1 data_store_memory; Handshake_2 data_store_memory; Filter data_store_memory; De_1 data_store_memory; De_2 data_store_memory; De_sum_1 data_store_memory; De_sum_2 data_store_memory
% Name: add_to_Send_Buffer
% Funktionalitäten
% Handshake-Message einfügen, wenn Status==1
% Delay-caculation-Message einfügen, wenn Status==2
% Sum-Delay-caculation-Message einfügen, wemm Status==3
% Nachrichten, die der Host senden möchte, einfügen, wenn Status==4

function add_to_Send_Buffer(status, lenS_1, lenS_2, to_send_signal, to_send_package)

global Send_Buffer_1
global Send_Buffer_2
global Address
global Address_1
global Address_2
global Handshake_1
global Handshake_2
global Filter
global De_1
global De_2
global De_sum_1
global De_sum_2

switch status
    case -2                         % Error Signal einrichten
        Filter(1,7) = 1;
    case 1                          % Handshake
        if((Filter(1,1) == 0) || ~Handshake_1)              % 103 not sent yet || Handshake_1 not finish yet
            check_1 = check_X(103, Address, Send_Buffer_1);          % check if there is a 103-Message in Send_Buffer_1
            if ~check_1
                Send_Buffer_1(lenS_1:lenS_1+7) = [Address, 0, 103, zeros(1,4), 102];
                Filter(1,1) = 1;                            % to remember, if 103 ist sent
            end
        end
        if((Filter(1,2) == 0) || ~Handshake_2)
            check_2 = check_X(103, Address, Send_Buffer_2);
            if ~check_2
                Send_Buffer_2(lenS_2:lenS_2+7) = [Address, 0, 103, zeros(1,4), 102];
                Filter(1,2) = 1;
            end
        end

        
    case 2                          % Delay time caculation
        if((Filter(1,3) == 0 ) || (De_1 <= 0))              % 105 not sent || De_1 not caculated yet
            check_1 = check_X(105, Address, Send_Buffer_1);
            if ~check_1
                Send_Buffer_1(lenS_1:lenS_1+7) = [Address, Address_2, 105, zeros(1,4), 102];
                Filter(1,3) = 1;
            end
        end
        if((Filter(1,4) == 0 ) || (De_2 <= 0))
            check_2 = check_X(105, Address, Send_Buffer_2);
            if ~check_2
                Send_Buffer_2(lenS_2:lenS_2+7) = [Address, Address_1, 105, zeros(1,4), 102];
                Filter(1,4) = 1;
            end
        end
        
    case 3                          % Sum_Delay caculation
        if((Filter(1,5) == 0 ) || (De_sum_1 <= 0))          % 107 not sent || De_sum_1 not caculated yet
            check_1 = check_X(107, Address, Send_Buffer_1);
            if ~check_1
                Send_Buffer_1(lenS_1:lenS_1+7) = [Address, Address, 107, zeros(1,4), 102];
                Filter(1,5) = 1;
            end
        end
        if((Filter(1,6) == 0 ) || (De_sum_2 <= 0))
            check_2 = check_X(107, Address, Send_Buffer_2);
            if ~check_2
                Send_Buffer_2(lenS_2:lenS_2+7) = [Address, Address, 107, zeros(1,4), 102];
                Filter(1,6) = 1;
            end
        end
        
    case 4                          % normal communication
        if to_send_signal
            check_1 = check_Y(to_send_package, Send_Buffer_1);
            check_2 = check_Y(to_send_package, Send_Buffer_2);
            if ~check_1
                Send_Buffer_1(lenS_1:lenS_1+21) = [to_send_package, 102];       % Attention!!!! 21 is the lenth of cariable 'wait_to_send'
            end
            if ~check_2
                Send_Buffer_2(lenS_2:lenS_2+21) = [to_send_package, 102];
            end
        end
end

end

function y = check_X(CMD, adr, Data)          % y: boolean; x: double, [1x100];

x = find(Data==CMD);
y = ~isempty(x);
if y
    y = y && (Data(1,x(1)-2) == adr);
end

end

function y = check_Y(data, Data)          % y: boolean; data: double, [1x6];

x = find(Data==data(3));        % CMD
y = ~isempty(x);
if y
    for i=1:length(x)
        if(isequal(Data(x(i)-2:x(i)+3),data(1:6)))
            y = true;
            break
        else
            y = false;
        end
    end
end

end

== matlab function Agent_ZP_Mananger/ZP_Mananger/Schnittstelle_1/Global_Var_Length ==
  data: len_Send_Buffer_1 output double size=1; len_Send_Buffer_2 output double size=1; len_Recv_Buffer output double size=1; len_Filter output double size=1; Send_Buffer_1 data_store_memory; Send_Buffer_2 data_store_memory; Recv_Buffer data_store_memory; Filter data_store_memory
% genutzte Länge der globale Variablen berechnen

function [len_Send_Buffer_1, len_Send_Buffer_2, len_Recv_Buffer, len_Filter] = Length
global Send_Buffer_1
global Send_Buffer_2
global Recv_Buffer
global Filter

a1 = find(Send_Buffer_1==102,1);
len_Send_Buffer_1 = a1(1);
a2 = find(Send_Buffer_2==102,1);
len_Send_Buffer_2 = a2(1);

len_Recv_Buffer = min(find(Recv_Buffer==0,150))-1;
len_Filter = min(find(Filter(2:20)==0,150));

end

== matlab function Agent_ZP_Mananger/ZP_Mananger/Schnittstelle_1/Recv_1 ==
  data: status input double size=1; clock input double size=1; lenS_1 input; lenS_2 input; lenR input; Rx_1_signal input boolean size=1; Rx_1_data input double size=[1 100]; recv_signal_1 output boolean; recv_package_1 output double size=[1 98]; Send_Buffer_1 data_store_memory; Send_Buffer_2 data_store_memory; T_send_1 data_store_memory; T_recv_1 data_store_memory; De_1 data_store_memory; De_sum_1 data_store_memory; Address data_store_memory; Recv_Buffer data_store_memory; Address_2 data_store_memory; Address_1 data_store_memory; De_sum_2 data_store_memory; Handshake_1 data_store_memory; De_2 data_store_memory; Handshake_2 data_store_memory; T_recv_2 data_store_memory; T_send_2 data_store_memory
% Name: Rx_1

% -------------------------------------------------------------------------------------
% Funktionalitäten:
% Im Init-Prozess
%   1. Handshake durch zu führen
%       103...Handshake ask --> 104 in Send_Buffer_2 additieren
%       104...Handshake answer --> Handshake success
%   2. Delay-Zeit berechnen
%       105...Delay begin --> 106 in Send_Buffer_2 additieren
%       106...Delay end --> Delay_Zeit berechnen
%   3. Sum-Delay-Zeit berechnen
%       107, Receiver = meine Addresse --> Sum_Delay_Zeit berechnen
%       107, Receiver ~= meine Addresse --> Daten in Send_Buffer_1 additieren
% Im normalen Prozess
%   4. Receiver = meine Addresse --> in Recv_Buffer additieren
%   5. Receiver = 255 --> Broadcast --> in Recv_Buffer && Send_Buffer_1 additieren
%   6. Receiver ~= meine Addresse --> in Send_Buffer_1 additieren

% -------------------------------------------------------------------------------------
% Input && Output
% status - status of 'Schnittstelle'
% clock - simulation time
% lenS_1/len_2/lenR - meaningful length of Send_Buffer_1/Send_Buffer_2/Recv_Buffer
% Rx_1_data - from Rx_1 received data
% recv_package_1 - data to send to chart or store in Send_Buffer_1
    % in Init-process, recv_package_1 need to be sent to chart
    % in normal-process, recv_package_1 need to garther all 'to be transmmited' datablock, and store in Send_Buffer_1

function [recv_signal_1, recv_package_1] = Rx_1(status, clock,lenS_1, lenS_2, lenR, Rx_1_signal, Rx_1_data)

global Send_Buffer_1
global Send_Buffer_2
global T_send_1
global T_recv_1
global De_1
%global De_2
global De_sum_1
global Address
global Address_1
%global Address_2
global Recv_Buffer
global Handshake_1

recv_signal_1 = false;
recv_package_1 = zeros(1,98);       % one datablock = [1x7]

lenr = 1;                           % path to write data into recv_package_1

if Rx_1_signal
    a = find(Rx_1_data==102,1);
    len = a(1);
    if ~isempty(len)
        mod_ = mod(len-2,7);
        len_ = ceil((len - 2) / 7);                                 % Round toward positive infinity
    end
    
	if ((mod_ == 0) && (len_ >= 1))                             % package contains at least one datablock
        switch status
            case 1                                              % Handshake
                for i=1:len_
                    switch Rx_1_data(7*i-3)                          % Da.cmd
                        case 103                                % Handshake ask --> send answer
                            check = check_X(104, Address, Send_Buffer_2);
                            if ((Rx_1_data(7*i-5) ~= 0) && (Rx_1_data(7*i-4) == 0) && ~Handshake_1 && ~check)
                                Address_1 = Rx_1_data(7*i-5);
                                Send_Buffer_2(lenS_2:lenS_2+7) = [Address, Address_1, 104, zeros(1,4), 102];
                            end
                        case 104                                % Handshake answer --> Handshake success --> no more send
                            if ((Rx_1_data(7*i-5) ~= 0) && (Rx_1_data(7*i-4) == Address) && ~Handshake_1)
                                Address_1 = Rx_1_data(7*i-5);        % Address of the Host in the Direction_1
                                recv_package_1(lenr:lenr+6) = Rx_1_data(7*i-5:7*i+1);    % [_,_,104,_,_,_,_] = [1x7]
                                lenr = lenr + 7;
                                recv_signal_1 = true;
                            end
                    end
                end

            case 2                                              % Delay_Time_Caculation
                for j=1:len_
                    switch Rx_1_data(7*j-3)                          % Da.cmd
                        case 103                                % Handshake ask --> send answer
                            check = check_X(104, Address, Send_Buffer_2);
                            if ((Rx_1_data(7*j-5) ~= 0) && (Rx_1_data(7*j-4) == 0) && ~Handshake_1 && ~check)
                                Address_1 = Rx_1_data(7*j-5);
                                Send_Buffer_2(lenS_2:lenS_2+7) = [Address, Address_1, 104, zeros(1,4), 102];
                            end
                        case 105                                % Delay ask --> send answer
                            check = check_X(106, Address, Send_Buffer_2);
                            if (isequal(Rx_1_data(7*j-5:7*j-4),[Address_1, Address]) && Handshake_1 && ~check) % check Sender & Receiver
                                Send_Buffer_2(lenS_2:lenS_2+7) = [Address, 0, 106, zeros(1,4), 102];
                            end
                        case 106                                % Delay answer --> caculate the time --> no more send
                            if ((isequal(Rx_1_data(7*j-5:7*j-3),[Address_1, Address, 106])) && (De_1 <= 0))
                                T_recv_1 = clock;
                                De_1 = T_recv_1 - T_send_1;
                                T_send_1 = 0;
                                T_recv_1 = 0;
                            end
                    end
                end

            case 3                                              % Sum_Delay_Caculation
                for h=1:len_
                    switch Rx_1_data(7*h-3)
                        case 103                                % Handshake ask --> send answer
                            check = check_X(104, Address, Send_Buffer_2);
                            if ((Rx_1_data(7*h-5) ~= 0) && (Rx_1_data(7*h-4) == 0) && ~Handshake_1 && ~check)
                                Address_1 = Rx_1_data(7*h-5);
                                Send_Buffer_2(lenS_2:lenS_2+7) = [Address, Address_1, 104, zeros(1,4), 102];
                            end
                        case 105                                % Delay ask --> send answer
                            check = check_X(106, Address, Send_Buffer_2);
                            if (isequal(Rx_1_data(7*h-5:7*h-4),[Address_1, Address]) && Handshake_1 && ~check) % check Sender & Receiver
                                Send_Buffer_2(lenS_2:lenS_2+7) = [Address, 0, 106, zeros(1,4), 102];
                            end   
                        case 107
                            if (isequal(Rx_1_data(7*h-5:7*h-4),[Address, Address]) && (De_sum_1 <= De_1))                   % Sum_Delay --> caculate the time --> no more send
                                T_recv_1 = clock;
                                De_sum_1 = T_recv_1 - T_send_1;
                                T_send_1 = 0;
                                T_recv_1 = 0;
                            elseif ((isequal(Rx_1_data(7*h-5),Rx_1_data(7*h-4))) && (Rx_1_data(7*h-5) ~= Address))
                                check = check_Y(Rx_1_data(7*h-5:7*h), recv_package_1) || check_Y(Rx_1_data(7*h-5:7*h), Send_Buffer_1);
                                if ~check
                                    recv_package_1(lenr:lenr+6) = Rx_1_data(7*h-5:7*h+1)';
                                    lenr = lenr + 7;
                                end
                            end
                    end
                end
                Send_Buffer_1(lenS_1:lenS_1+lenr-1) = [recv_package_1(1:lenr-1),102];           % 前提：lenS更新速度比当前更新快

            case 4                                               % normal communication between all Hosts
                for k=1:len_
                    switch Rx_1_data(7*k-3)
                        case 103                                % Handshake ask --> send answer
                            check = check_X(104, Address, Send_Buffer_2);
                            if ((Rx_1_data(7*k-5) ~= 0) && (Rx_1_data(7*k-4) == 0) && ~Handshake_1 && ~check)
                                Address_1 = Rx_1_data(7*k-5);
                                Send_Buffer_2(lenS_2:lenS_2+7) = [Address, Address_1, 104, zeros(1,4), 102];
                            end
                        case 105                                % Delay ask --> send answer
                            check = check_X(106, Address, Send_Buffer_2);
                            if (isequal(Rx_1_data(7*k-5:7*k-4),[Address_1, Address]) && Handshake_1 && ~check) % check Sender & Receiver
                                Send_Buffer_2(lenS_2:lenS_2+7) = [Address, 0, 106, zeros(1,4), 102];
                            end
                        case 107
                            if ((isequal(Rx_1_data(7*k-5),Rx_1_data(7*k-4))) && (Rx_1_data(7*k-5) ~= Address))
                                check = check_Y(Rx_1_data(7*k-5:7*k), recv_package_1) || check_Y(Rx_1_data(7*k-5:7*k), Send_Buffer_1);
                                if ~check
                                    recv_package_1(lenr:lenr+6) = Rx_1_data(7*k-5:7*k+1)';
                                    lenr = lenr + 7;
                                end
                            end
                        otherwise
                            if ((Rx_1_data(7*k-5) ~= Address) && (Rx_1_data(7*k-4) == Address))   % Datablock sent to me --> store in Recv_Buffer
                                check = check_Y(Rx_1_data(7*k-5:7*k), Recv_Buffer');
                                if ~check
                                    Recv_Buffer(lenR+1,:) = Rx_1_data(7*k-5:7*k+1);
                                end
                            elseif ((Rx_1_data(7*k-5) ~=Address) && (Rx_1_data(7*k-4) == 255))    % Datablock is as a Broadcast --> store in Recv_Buffer && Send_Buffer_1
                                check = check_Y(Rx_1_data(7*k-5:7*k), Recv_Buffer');
                                if ~check
                                    Recv_Buffer(lenR+1,:) = Rx_1_data(7*k-5:7*k+1);
                                end
                                check = check_Y(Rx_1_data(7*k-5:7*k), recv_package_1) || check_Y(Rx_1_data(7*k-5:7*k), Send_Buffer_1);
                                if ~check
                                    recv_package_1(lenr:lenr+6) = Rx_1_data(7*k-5:7*k+1)';
                                    lenr = lenr + 7;
                                end
                            elseif ((Rx_1_data(7*k-4) ~= Address) && (Rx_1_data(7*k-4) ~= 255))   % Datablock not sent to me --> to transmmit --> store in Send_Buffer_1
                                check = check_Y(Rx_1_data(7*k-5:7*k), recv_package_1) || check_Y(Rx_1_data(7*k-5:7*k), Send_Buffer_1);
                                if ~check
                                    recv_package_1(lenr:lenr+6) = Rx_1_data(7*k-5:7*k+1)';
                                    lenr = lenr + 7;
                                end
                            end
                    end
                end
                Send_Buffer_1(lenS_1:lenS_1+lenr-1) = [recv_package_1(1:lenr-1),102];
        end
	elseif mod_ ~= 0
        fprintf("Eroor: Package length not avalueable!");
	end
end

end

% check_X: to check if Data contains a Datablock with CMD and adr
function y = check_X(CMD, adr, Data)          % y: boolean; x: double, [1x100];

x = find(Data==CMD);
y = (~isempty(x));

if y
    y = y && (Data(1,x(1)-2) == adr);
end

end

% check_Y: to check if Data contains data
function y = check_Y(data, Data)          % y: boolean; data: double, [1x6];

x = find(Data==data(3));
y = (~isempty(x));
if y
    for i=1:length(x)
        if(isequal(Data(x(i)-2:x(i)+3),data))
            y = true;
            break
        else
            y = false;
        end
    end
end

end
